simulink model "ADU_Integration_R2014a_simulation"  (R2014a)
settings: Solver=FixedStepDiscrete  StartTime=285  StopTime=300  FixedStep=0.01  RelTol=1e-3
PostLoadFcn:
  | , if any(exist('dsrtsu_mdlpostloadfcn', 'file') == [2, 3, 6]), try dsrtsu_mdlpostloadfcn('Execute', bdroot); catch fprintf('Error in PostLoadFcn (dsrtsu_mdlpostloadfcn) for model "%s":\n %s\n', bdroot, lasterr); end, end,
InitFcn:
  | load 'data/chi2_dat';
  | load 'data/Line_struct';
  | load 'data/innerLNM_1';
  | load 'data/middleLNM_2';
  | load 'data/outerLNM_1';
  | load 'data/landmarks_patac_schimmel_ccw';
  | load 'data/patac_navi_array';
  | load 'data/sensor';
  | load 'data/map_struct';
  | addpath map_src
  | Integration_Parameter;
  | load 'TestData_001';
values from neighbouring files (symbols this model uses):
  TestData_001 =     [TestData_001.mat]
undefined symbols (not defined in the file or in its folder): chi2_dat, innerLNM_1, landmarks_patac_schimmel_ccw, middleLNM_2, outerLNM_1, patac_navi_array
libraries: simulink x36, rtican x1
(part 3 of 22)

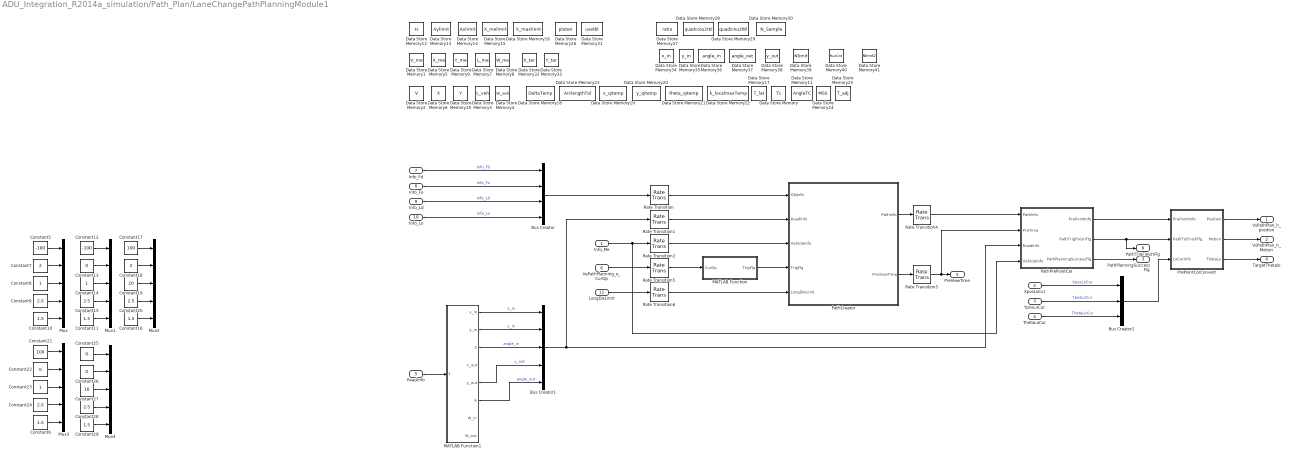
== system ADU_Integration_R2014a_simulation/Path_Plan/LaneChangePathPlanningModule1 ==
  Info_Me : Inport
  XposLoCur : Inport  Port=2
  YposLoCur : Inport  Port=3
  ThetaLoCur : Inport  Port=4
  RoadInfo : Inport  Port=5
  VePathPlanning_e_CurOp : Inport  Port=6
  Info_Fd : Inport  Port=7
  Info_Fo : Inport  Port=8
  Info_Ld : Inport  Port=9
  Info_Lo : Inport  Port=10
  LongDisLimit : Inport  Port=11
  Bus Creator : BusCreator  Inputs=4
  Bus Creator1 : BusCreator  Inputs=5
  Bus Creator2 : BusCreator  Inputs=3
  Constant{6,10..11,16,29} (5 alike) : Constant  Value=1.5
  Constant12 : Constant  Value=-100
  Constant{13,22,25..26} (4 alike) : Constant  Value=0
  Constant14 : Constant
  Constant{9,15,20,24,28} (5 alike) : Constant  Value=2.5
  Constant17 : Constant  Value=100
  Constant18 : Constant  Value=2
  Constant19 : Constant  Value=20
  Constant21 : Constant  Value=100
  Constant23 : Constant
  Constant27 : Constant  Value=10
  Constant5 : Constant  Value=-100
  Constant7 : Constant  Value=2
  Constant8 : Constant
  Data Store Memory : DataStoreMemory  DataStoreName=Tc  ReadBeforeWriteMsg=warning  WriteAfterWriteMsg=warning  WriteAfterReadMsg=warning  InitialValue=[0 0 0 0]  ShowAdditionalParam=off  OutDataTypeStr=double
  Data Store Memory1 : DataStoreMemory  DataStoreName=V_me  ReadBeforeWriteMsg=warning  WriteAfterWriteMsg=warning  WriteAfterReadMsg=warning  ShowAdditionalParam=off  OutDataTypeStr=double
  Data Store Memory10 : DataStoreMemory  DataStoreName=Y  ReadBeforeWriteMsg=warning  WriteAfterWriteMsg=warning  WriteAfterReadMsg=warning  InitialValue=[0 0 0 0]  ShowAdditionalParam=off  OutDataTypeStr=double
  Data Store Memory11 : DataStoreMemory  DataStoreName=AngleTC  ReadBeforeWriteMsg=warning  WriteAfterWriteMsg=warning  WriteAfterReadMsg=warning  InitialValue=[0 0 0 0]  ShowAdditionalParam=off  OutDataTypeStr=double
  Data Store Memory12 : DataStoreMemory  DataStoreName=H  ReadBeforeWriteMsg=warning  WriteAfterWriteMsg=warning  WriteAfterReadMsg=warning  ShowAdditionalParam=off  OutDataTypeStr=double
  Data Store Memory13 : DataStoreMemory  DataStoreName=Aylimit  ReadBeforeWriteMsg=warning  WriteAfterWriteMsg=warning  WriteAfterReadMsg=warning  ShowAdditionalParam=off  OutDataTypeStr=double
  Data Store Memory14 : DataStoreMemory  DataStoreName=Axlimit  ReadBeforeWriteMsg=warning  WriteAfterWriteMsg=warning  WriteAfterReadMsg=warning  ShowAdditionalParam=off  OutDataTypeStr=double
  Data Store Memory15 : DataStoreMemory  DataStoreName=X_melimit  ReadBeforeWriteMsg=warning  WriteAfterWriteMsg=warning  WriteAfterReadMsg=warning  ShowAdditionalParam=off  OutDataTypeStr=double
  Data Store Memory16 : DataStoreMemory  DataStoreName=k_maxlimit  ReadBeforeWriteMsg=warning  WriteAfterWriteMsg=warning  WriteAfterReadMsg=warning  ShowAdditionalParam=off  OutDataTypeStr=double
  Data Store Memory17 : DataStoreMemory  DataStoreName=T_lat  ReadBeforeWriteMsg=warning  WriteAfterWriteMsg=warning  WriteAfterReadMsg=warning  ShowAdditionalParam=off  OutDataTypeStr=double
  Data Store Memory18 : DataStoreMemory  DataStoreName=DeltaTemp  ReadBeforeWriteMsg=warning  WriteAfterWriteMsg=warning  WriteAfterReadMsg=warning  InitialValue=[0 0]  ShowAdditionalParam=off  OutDataTypeStr=double
  Data Store Memory19 : DataStoreMemory  DataStoreName=x_qitemp  ReadBeforeWriteMsg=warning  WriteAfterWriteMsg=warning  WriteAfterReadMsg=warning  ShowAdditionalParam=off  OutDataTypeStr=double
  Data Store Memory2 : DataStoreMemory  DataStoreName=V  ReadBeforeWriteMsg=warning  WriteAfterWriteMsg=warning  WriteAfterReadMsg=warning  InitialValue=[0 0 0 0]  ShowAdditionalParam=off  OutDataTypeStr=double
  Data Store Memory20 : DataStoreMemory  DataStoreName=y_qitemp  ReadBeforeWriteMsg=warning  WriteAfterWriteMsg=warning  WriteAfterReadMsg=warning  ShowAdditionalParam=off  OutDataTypeStr=double
  Data Store Memory21 : DataStoreMemory  DataStoreName=theta_qitemp  ReadBeforeWriteMsg=warning  WriteAfterWriteMsg=warning  WriteAfterReadMsg=warning  ShowAdditionalParam=off  OutDataTypeStr=double
  Data Store Memory22 : DataStoreMemory  DataStoreName=k_localmaxTemp  ReadBeforeWriteMsg=warning  WriteAfterWriteMsg=warning  WriteAfterReadMsg=warning  InitialValue=[0 0]  ShowAdditionalParam=off  OutDataTypeStr=double
  Data Store Memory23 : DataStoreMemory  DataStoreName=ArclengthTol  ReadBeforeWriteMsg=warning  WriteAfterWriteMsg=warning  WriteAfterReadMsg=warning  InitialValue=[0 0]  ShowAdditionalParam=off  OutDataTypeStr=double
  Data Store Memory24 : DataStoreMemory  DataStoreName=MSS  ReadBeforeWriteMsg=warning  WriteAfterWriteMsg=warning  WriteAfterReadMsg=warning  InitialValue=[0 0 0 0]  ShowAdditionalParam=off  OutDataTypeStr=double
  Data Store Memory25 : DataStoreMemory  DataStoreName=T_adj  ReadBeforeWriteMsg=warning  WriteAfterWriteMsg=warning  WriteAfterReadMsg=warning  ShowAdditionalParam=off  OutDataTypeStr=double
  Data Store Memory26 : DataStoreMemory  DataStoreName=ploten  ReadBeforeWriteMsg=warning  WriteAfterWriteMsg=warning  WriteAfterReadMsg=warning  ShowAdditionalParam=off  OutDataTypeStr=double
  Data Store Memory27 : DataStoreMemory  DataStoreName=ratio  ReadBeforeWriteMsg=warning  WriteAfterWriteMsg=warning  WriteAfterReadMsg=warning  ShowAdditionalParam=off  OutDataTypeStr=double
  Data Store Memory28 : DataStoreMemory  DataStoreName=quadcosu2tbl  ReadBeforeWriteMsg=warning  WriteAfterWriteMsg=warning  WriteAfterReadMsg=warning  InitialValue=zeros(1,356)  ShowAdditionalParam=off  OutDataTypeStr=double
  Data Store Memory29 : DataStoreMemory  DataStoreName=quadsinu2tbl  ReadBeforeWriteMsg=warning  WriteAfterWriteMsg=warning  WriteAfterReadMsg=warning  InitialValue=zeros(1,356)  ShowAdditionalParam=off  OutDataTypeStr=double
  Data Store Memory3 : DataStoreMemory  DataStoreName=L_veh  ReadBeforeWriteMsg=warning  WriteAfterWriteMsg=warning  WriteAfterReadMsg=warning  InitialValue=[0 0 0 0]  ShowAdditionalParam=off  OutDataTypeStr=double
  Data Store Memory30 : DataStoreMemory  DataStoreName=N_Sample  ReadBeforeWriteMsg=warning  WriteAfterWriteMsg=warning  WriteAfterReadMsg=warning  ShowAdditionalParam=off  OutDataTypeStr=double
  Data Store Memory31 : DataStoreMemory  DataStoreName=usetbl  ReadBeforeWriteMsg=warning  WriteAfterWriteMsg=warning  WriteAfterReadMsg=warning  ShowAdditionalParam=off  OutDataTypeStr=double
  Data Store Memory32 : DataStoreMemory  DataStoreName=X_tar  ReadBeforeWriteMsg=warning  WriteAfterWriteMsg=warning  WriteAfterReadMsg=warning  ShowAdditionalParam=off  OutDataTypeStr=double
  Data Store Memory33 : DataStoreMemory  DataStoreName=Y_tar  ReadBeforeWriteMsg=warning  WriteAfterWriteMsg=warning  WriteAfterReadMsg=warning  ShowAdditionalParam=off  OutDataTypeStr=double
  Data Store Memory34 : DataStoreMemory  DataStoreName=x_in  ReadBeforeWriteMsg=warning  WriteAfterWriteMsg=warning  WriteAfterReadMsg=warning  ShowAdditionalParam=off  OutDataTypeStr=double
  Data Store Memory35 : DataStoreMemory  DataStoreName=y_in  ReadBeforeWriteMsg=warning  WriteAfterWriteMsg=warning  WriteAfterReadMsg=warning  ShowAdditionalParam=off  OutDataTypeStr=double
  Data Store Memory36 : DataStoreMemory  DataStoreName=angle_in  ReadBeforeWriteMsg=warning  WriteAfterWriteMsg=warning  WriteAfterReadMsg=warning  ShowAdditionalParam=off  OutDataTypeStr=double
  Data Store Memory37 : DataStoreMemory  DataStoreName=angle_out  ReadBeforeWriteMsg=warning  WriteAfterWriteMsg=warning  WriteAfterReadMsg=warning  ShowAdditionalParam=off  OutDataTypeStr=double
  Data Store Memory38 : DataStoreMemory  DataStoreName=y_out  ReadBeforeWriteMsg=warning  WriteAfterWriteMsg=warning  WriteAfterReadMsg=warning  ShowAdditionalParam=off  OutDataTypeStr=double
  Data Store Memory39 : DataStoreMemory  DataStoreName=Nlimit  ReadBeforeWriteMsg=warning  WriteAfterWriteMsg=warning  WriteAfterReadMsg=warning  ShowAdditionalParam=off  OutDataTypeStr=double
  Data Store Memory4 : DataStoreMemory  DataStoreName=W_veh  ReadBeforeWriteMsg=warning  WriteAfterWriteMsg=warning  WriteAfterReadMsg=warning  InitialValue=[0 0 0 0]  ShowAdditionalParam=off  OutDataTypeStr=double
  Data Store Memory40 : DataStoreMemory  DataStoreName=RunCnt  ReadBeforeWriteMsg=warning  WriteAfterWriteMsg=warning  WriteAfterReadMsg=warning  InitialValue=[0 0 0 0]  ShowAdditionalParam=off  OutDataTypeStr=double
  Data Store Memory41 : DataStoreMemory  DataStoreName=Nlimit2  ReadBeforeWriteMsg=warning  WriteAfterWriteMsg=warning  WriteAfterReadMsg=warning  ShowAdditionalParam=off  OutDataTypeStr=double
  Data Store Memory5 : DataStoreMemory  DataStoreName=X_me  ReadBeforeWriteMsg=warning  WriteAfterWriteMsg=warning  WriteAfterReadMsg=warning  ShowAdditionalParam=off  OutDataTypeStr=double
  Data Store Memory6 : DataStoreMemory  DataStoreName=X  ReadBeforeWriteMsg=warning  WriteAfterWriteMsg=warning  WriteAfterReadMsg=warning  InitialValue=[0 0 0 0]  ShowAdditionalParam=off  OutDataTypeStr=double
  Data Store Memory7 : DataStoreMemory  DataStoreName=L_me  ReadBeforeWriteMsg=warning  WriteAfterWriteMsg=warning  WriteAfterReadMsg=warning  ShowAdditionalParam=off  OutDataTypeStr=double
  Data Store Memory8 : DataStoreMemory  DataStoreName=W_me  ReadBeforeWriteMsg=warning  WriteAfterWriteMsg=warning  WriteAfterReadMsg=warning  ShowAdditionalParam=off  OutDataTypeStr=double
  Data Store Memory9 : DataStoreMemory  DataStoreName=Y_me  ReadBeforeWriteMsg=warning  WriteAfterWriteMsg=warning  WriteAfterReadMsg=warning  ShowAdditionalParam=off  OutDataTypeStr=double
  MATLAB Function : MATLAB Function  TreatAsAtomicUnit=on
      settings: PermitHierarchicalResolution=ParametersOnly
  MATLAB Function1 : MATLAB Function  TreatAsAtomicUnit=on
      settings: PermitHierarchicalResolution=ParametersOnly
  Mux{,1..4} (5 alike) : Mux  Inputs=5
  PathCreator : Subsystem  TreatAsAtomicUnit=on  SystemSampleTime=0.02
  PathPrePointCal : Subsystem  TreatAsAtomicUnit=on
  PrePointCorConvert : Subsystem  TreatAsAtomicUnit=on
  Rate Transition{,1..2,5..6} (5 alike) : RateTransition  OutPortSampleTime=0.02
  Rate Transition3 : RateTransition  OutPortSampleTime=0.01
  Rate Transition4 : RateTransition  OutPortSampleTime=0.01
  VsPathPlan_h_position : Outport
  VsPathPlan_h_Motion : Outport  Port=2
  PathPlanningSuccessFlg : Outport  Port=3
  TargetThetalo : Outport  Port=4
  PreViewTime : Outport  Port=5
  PathTrigFinishFlg : Outport  Port=6
  wires:
  MATLAB Function/1(TrigFlg) -> PathCreator/4(TrigFlg)
  Rate Transition5/1 -> MATLAB Function/1(CurOp)
  VePathPlanning_e_CurOp/1 -> Rate Transition5/1
  Rate Transition3/1 -> PreViewTime/1, PathPrePointCal/2(PreTime)
  PathPrePointCal/2(PathTrigFinishFlg) -> PrePointCorConvert/2(PathTrjFinishFlg), PathTrigFinishFlg/1
  PathCreator/2(PreViewTime) -> Rate Transition3/1
  PathPrePointCal/3(PathPlanningSuccessFlg) -> PathPlanningSuccessFlg/1
  Rate Transition4/1 -> PathPrePointCal/1(PathInfo)
  Rate Transition2/1 -> PathCreator/3(VehicleInfo)
  PathCreator/1(PathInfo) -> Rate Transition4/1
  Rate Transition1/1 -> PathCreator/2(RoadInfo)
  Rate Transition/1 -> PathCreator/1(ObjInfo)
  PrePointCorConvert/3(ThetaLo) -> TargetThetalo/1
  PrePointCorConvert/2(Motion) -> VsPathPlan_h_Motion/1
  PrePointCorConvert/1(Position) -> VsPathPlan_h_position/1
  Bus Creator2/1 -> PrePointCorConvert/3(LoCorInfo)
  PathPrePointCal/1(PrePointInfo) -> PrePointCorConvert/1(PrePointInfo)
  ThetaLoCur/1 -> Bus Creator2/3  "ThetaLoCur"
  YposLoCur/1 -> Bus Creator2/2  "YposLoCur"
  XposLoCur/1 -> Bus Creator2/1  "XposLoCur"
  Bus Creator1/1 -> Rate Transition1/1, PathPrePointCal/3(RoadInfo)
  MATLAB Function1/6(angle_out) -> Bus Creator1/5  "angle_out"
  MATLAB Function1/5(y_out) -> Bus Creator1/4  "y_out"
  MATLAB Function1/3(angle_in) -> Bus Creator1/3  "angle_in"
  MATLAB Function1/2(y_in) -> Bus Creator1/2  "y_in"
  MATLAB Function1/1(x_in) -> Bus Creator1/1  "x_in"
  Bus Creator/1 -> Rate Transition/1
  Info_Lo/1 -> Bus Creator/4  "Info_Lo"
  Info_Ld/1 -> Bus Creator/3  "Info_Ld"
  Info_Fo/1 -> Bus Creator/2  "Info_Fo"
  Info_Fd/1 -> Bus Creator/1  "Info_Fd"
  Info_Me/1 -> PathPrePointCal/4(VehicleInfo), Rate Transition2/1
  Constant25/1 -> Mux4/1
  Constant21/1 -> Mux3/1
  Constant27/1 -> Mux4/3
  Constant29/1 -> Mux4/5
  Constant28/1 -> Mux4/4
  Constant26/1 -> Mux4/2
  Constant23/1 -> Mux3/3
  Constant6/1 -> Mux3/5
  Constant24/1 -> Mux3/4
  Constant22/1 -> Mux3/2
  Constant5/1 -> Mux/1
  Constant19/1 -> Mux2/3
  Constant16/1 -> Mux2/5
  Constant20/1 -> Mux2/4
  Constant18/1 -> Mux2/2
  Constant17/1 -> Mux2/1
  Constant14/1 -> Mux1/3
  Constant11/1 -> Mux1/5
  Constant15/1 -> Mux1/4
  Constant13/1 -> Mux1/2
  Constant12/1 -> Mux1/1
  Constant8/1 -> Mux/3
  Constant10/1 -> Mux/5
  Constant9/1 -> Mux/4
  Constant7/1 -> Mux/2
  RoadInfo/1 -> MATLAB Function1/1(RoadInfo)
  LongDisLimit/1 -> Rate Transition6/1
  Rate Transition6/1 -> PathCreator/5(LongDisLimit)

== system ADU_Integration_R2014a_simulation/Path_Plan/PathArbModule ==
  VsPathPlan_h_InterSecposition : Inport
  VsPathPlan_h_InterSecMotion : Inport  Port=2
  VePathPlan_e_InterPPSucFlg : Inport  Port=3
  TargetThetaLoInter : Inport  Port=4
  PreviewTimeInter : Inport  Port=5
  PathTrigFinishFlgInter : Inport  Port=6
  VsPathPlan_h_LCposition : Inport  Port=7
  VsPathPlan_h_LCMotion : Inport  Port=8
  VePathPlan_e_LCPPSucFlg : Inport  Port=9
  TargetThetaLoLC : Inport  Port=10
  PreviewTimeLC : Inport  Port=11
  PathTrigFinishFlgLC : Inport  Port=12
  VePathPlan_e_OutputSelection : Inport  Port=13
  Bus Creator : BusCreator  Inputs=6
  Bus Creator1 : BusCreator  Inputs=6
  Bus Selector : BusSelector  OutputSignals=VsPathPlan_h_position,VsPathPlan_h_Motion,VePathPlan_e_PPSucFlg,TargetThetaLo,PreviewTime,PathTrigFinishFlg
  Switch : Switch  Threshold=0.5
  VsPathPlan_h_position : Outport
  VsPathPlan_h_Motion : Outport  Port=2
  VePathPlan_b_InChargFlg : Outport  Port=3
  TargetThetaLo : Outport  Port=4
  PreviewTime : Outport  Port=5
  PathTrigFinishFlg : Outport  Port=6
  wires:
  Bus Selector/6 -> PathTrigFinishFlg/1  "<PathTrigFinishFlg>"
  PathTrigFinishFlgInter/1 -> Bus Creator1/6  "PathTrigFinishFlg"
  PathTrigFinishFlgLC/1 -> Bus Creator/6  "PathTrigFinishFlg"
  VePathPlan_e_OutputSelection/1 -> Switch/2
  PreviewTimeLC/1 -> Bus Creator/5  "PreviewTime"
  PreviewTimeInter/1 -> Bus Creator1/5  "PreviewTime"
  Bus Selector/1 -> VsPathPlan_h_position/1  "<VsPathPlan_h_position>"
  Bus Selector/2 -> VsPathPlan_h_Motion/1  "<VsPathPlan_h_Motion>"
  Bus Selector/3 -> VePathPlan_b_InChargFlg/1  "<VePathPlan_e_PPSucFlg>"
  Bus Selector/4 -> TargetThetaLo/1  "<TargetThetaLo>"
  Bus Selector/5 -> PreviewTime/1  "<PreviewTime>"
  Switch/1 -> Bus Selector/1
  Bus Creator1/1 -> Switch/3
  VsPathPlan_h_InterSecposition/1 -> Bus Creator1/1  "VsPathPlan_h_position"
  VsPathPlan_h_InterSecMotion/1 -> Bus Creator1/2  "VsPathPlan_h_Motion"
  VePathPlan_e_InterPPSucFlg/1 -> Bus Creator1/3  "VePathPlan_e_PPSucFlg"
  TargetThetaLoInter/1 -> Bus Creator1/4  "TargetThetaLo"
  Bus Creator/1 -> Switch/1
  VsPathPlan_h_LCposition/1 -> Bus Creator/1  "VsPathPlan_h_position"
  VsPathPlan_h_LCMotion/1 -> Bus Creator/2  "VsPathPlan_h_Motion"
  VePathPlan_e_LCPPSucFlg/1 -> Bus Creator/3  "VePathPlan_e_PPSucFlg"
  TargetThetaLoLC/1 -> Bus Creator/4  "TargetThetaLo"

== system ADU_Integration_R2014a_simulation/Path_Plan/SceneSelectionModule ==
  Sur_LandmarkIdList : Inport
  Veh_State : Inport  Port=2
  Object_Info : Inport  Port=3
  Sur_ObjectId_List : Inport  Port=4
  Landmark_Info : Inport  Port=5
  Navi_LandmarkIdList : Inport  Port=6
  EgoLane_Index : Inport  Port=7
  OperationFinishFlg : Inport  Port=8
  ObjSelect : MATLAB Function  TreatAsAtomicUnit=on
      settings: PermitHierarchicalResolution=ParametersOnly
  OpSchedule : MATLAB Function  TreatAsAtomicUnit=on
      settings: PermitHierarchicalResolution=ParametersOnly
  Info_Me : Outport
  Info_Fd : Outport  Port=2
  Info_Fo : Outport  Port=3
  Info_Ld : Outport  Port=4
  Info_Lo : Outport  Port=5
  CurOp : Outport  Port=6
  LongDisLimit : Outport  Port=7
  RoadInfo : Outport  Port=8
  wires:
  OpSchedule/2(OperationLongDislimit) -> LongDisLimit/1
  OperationFinishFlg/1 -> OpSchedule/1(OperationFinishFlg)
  OpSchedule/1(Curoperation) -> CurOp/1
  ObjSelect/1(Info_Fd) -> Info_Fd/1, OpSchedule/6(Info_Fd)
  ObjSelect/2(Info_Fo) -> Info_Fo/1, OpSchedule/7(Info_Fo)
  ObjSelect/4(Info_Lo) -> Info_Lo/1, OpSchedule/9(Info_Lo)
  ObjSelect/3(Info_Ld) -> Info_Ld/1, OpSchedule/8(Info_Ld)
  ObjSelect/5(Info_Me) -> Info_Me/1, OpSchedule/10(Info_Me)
  Object_Info/1 -> ObjSelect/4(Object_Info)
  Veh_State/1 -> ObjSelect/2(Veh_State)
  Sur_ObjectId_List/1 -> ObjSelect/3(Sur_ObjectId_List)
  EgoLane_Index/1 -> OpSchedule/5(EgoLane_Index), ObjSelect/1(EgoLane_Index)
  Landmark_Info/1 -> OpSchedule/2(Landmark_Info)
  Sur_LandmarkIdList/1 -> OpSchedule/3(Sur_LandmarkIdList)
  Navi_LandmarkIdList/1 -> OpSchedule/4(Navi_LandmarkIdList)
  OpSchedule/4(RoadInfo) -> RoadInfo/1

== system ADU_Integration_R2014a_simulation/Fusion_Model/Fusion_Block/Fus_Header_Gen ==
  Target_Num : Inport
  Bus Creator1 : BusCreator  Inputs=7
  CameraValid : Constant
  ESRValid : Constant
  LFSRRValid : Constant
  LRSRRValid1 : Constant
  RFSRRValid1 : Constant
  RRSRRValid2 : Constant
  Fus_Header : Outport
  wires:
  ESRValid/1 -> Bus Creator1/2  "ESRValid"
  LFSRRValid/1 -> Bus Creator1/3  "LFSRRValid"
  CameraValid/1 -> Bus Creator1/1  "CameraValid"
  RFSRRValid1/1 -> Bus Creator1/4  "RFSRRValid"
  RRSRRValid2/1 -> Bus Creator1/6  "RRSRRValid"
  Bus Creator1/1 -> Fus_Header/1
  LRSRRValid1/1 -> Bus Creator1/5  "LRSRRValid"
  Target_Num/1 -> Bus Creator1/7  "Total_Targ_Num"

== system ADU_Integration_R2014a_simulation/Fusion_Model/Fusion_Block/Global_Fusion ==
  From SideFusion : Inport
  From Sensor : Inport  Port=2
  Bus Selector1 : BusSelector  OutputSignals=Vision_Target[25X8]
  Bus Selector2 : BusSelector  OutputSignals=ESR_Data[64X4]
  Curve_Radius[m] : Subsystem
  ESR_TemporalAlig : Stateflow chart  TreatAsAtomicUnit=on
      settings: PermitHierarchicalResolution=ParametersOnly
  Fusion_Center : Stateflow chart  TreatAsAtomicUnit=on
      settings: PermitHierarchicalResolution=ParametersOnly
  Mux : Mux  Inputs=3
  Rate Transition1 : RateTransition  Deterministic=off
  Rate Transition2 : RateTransition  Deterministic=off
  Rate Transition3 : RateTransition  Deterministic=off
  Terminator1 : Terminator
  Terminator3 : Terminator
  GlobalFusOut[127X26] : Outport
  Total_TargetNum : Outport  Port=2
  wires:
  From Sensor/1 -> Bus Selector1/1, Bus Selector2/1
  Bus Selector2/1 -> ESR_TemporalAlig/1(ESR_Input)  "<ESR_Data[64X4]>"
  [ESRcal] -> ESR_TemporalAlig/Trigger
  [CameraCal] -> Mux/1
  [SRRCal] -> Mux/2
  ESR_TemporalAlig/1(ESR_Output) -> Fusion_Center/1(ESRData)
  Fusion_Center/1(FusDataOut) -> GlobalFusOut[127X26]/1
  Fusion_Center/2(Num_Trg) -> Total_TargetNum/1
  Bus Selector1/1 -> Fusion_Center/2(CameraData)  "<Vision_Target[25X8]>"
  From SideFusion/1 -> Fusion_Center/3(SRRData)
  Curve_Radius[m]/1(Curve_Radius[m]) -> Fusion_Center/4(Path_Radius)
  [ESRcal] -> Mux/3
  Mux/1 -> Fusion_Center/Trigger
  Fusion_Center/3(RollCount) -> Terminator3/1
  ESR_TemporalAlig/2(RollCount) -> Terminator1/1
  [CameraTime] -> Rate Transition1/1
  Rate Transition1/1 -> Fusion_Center/7(Camera_RxTime)
  [ESRTime] -> Rate Transition2/1
  Rate Transition2/1 -> Fusion_Center/5(ESR_RxTime)
  [LFSRRTime] -> Rate Transition3/1
  Rate Transition3/1 -> Fusion_Center/6(SRR_RxTime)

== system ADU_Integration_R2014a_simulation/Fusion_Model/Fusion_Block/Side_Fusion ==
  From Sensor : Inport
  Bus Selector2 : BusSelector  OutputSignals=LF_SRR_Data[10X5],RF_SRR_Data[10X5],LR_SRR_Data[10X5],RR_SRR_Data[10X5]
  LF_SRR_CoordinateAlig : Stateflow chart  TreatAsAtomicUnit=on
      settings: PermitHierarchicalResolution=ParametersOnly
  LR_SRR_CoordinateAlig : Stateflow chart  TreatAsAtomicUnit=on
      settings: PermitHierarchicalResolution=ParametersOnly
  Mux : Mux
  RF_SRR_CoordinateAlig : Stateflow chart  TreatAsAtomicUnit=on
      settings: PermitHierarchicalResolution=ParametersOnly
  RR_SRR_CoordinateAlig : Stateflow chart  TreatAsAtomicUnit=on
      settings: PermitHierarchicalResolution=ParametersOnly
  Rate Transition{1..4} (4 alike) : RateTransition  Deterministic=off
  SRR_Data_Out : Stateflow chart  TreatAsAtomicUnit=on
      settings: PermitHierarchicalResolution=ParametersOnly
  Side_Fusion : Stateflow chart  TreatAsAtomicUnit=on
      settings: PermitHierarchicalResolution=ParametersOnly
  SideFus_Output[40X4] : Outport
  SideRadar_RawData[40X4] : Outport  Port=2
  tag scope: SRRCal=global
  wires:
  Bus Selector2/1 -> LF_SRR_CoordinateAlig/1(LFSRR_Input)  "<LF_SRR_Data[10X5]>"
  Bus Selector2/2 -> RF_SRR_CoordinateAlig/1(RFSRR_Input)  "<RF_SRR_Data[10X5]>"
  Bus Selector2/3 -> LR_SRR_CoordinateAlig/1(LRSRR_Input)  "<LR_SRR_Data[10X5]>"
  Bus Selector2/4 -> RR_SRR_CoordinateAlig/1(RRSRR_Input)  "<RR_SRR_Data[10X5]>"
  LF_SRR_CoordinateAlig/1(LFSRR_Output) -> Side_Fusion/1(LFSRR_Input), SRR_Data_Out/1(LFSRR_Input)
  RF_SRR_CoordinateAlig/1(RFSRR_Output) -> Side_Fusion/3(RFSRR_Input), SRR_Data_Out/2(RFSRR_Input)
  LR_SRR_CoordinateAlig/1(LRSRR_Output) -> Side_Fusion/5(LRSRR_Input), SRR_Data_Out/3(LRSRR_Input)
  Side_Fusion/1(SideFusOut) -> SideFus_Output[40X4]/1
  From Sensor/1 -> Bus Selector2/1
  [LFSRRcal] -> LF_SRR_CoordinateAlig/Trigger
  [LRSRRcal] -> LR_SRR_CoordinateAlig/Trigger
  [RRSRRcal] -> RR_SRR_CoordinateAlig/Trigger
  LF_SRR_CoordinateAlig/2(SideFusion()) -> [LFSRRUpdate]
  RF_SRR_CoordinateAlig/2(SideFusion()) -> [RFSRRUpdate]
  LR_SRR_CoordinateAlig/2(SideFusion()) -> [LRSRRUpdate]
  RR_SRR_CoordinateAlig/2(SideFusion()) -> [RRSRRUpdate]
  [LFSRRUpdate] -> Mux/1
  [RFSRRUpdate] -> Mux/2
  [LRSRRUpdate] -> Mux/3
  [RRSRRUpdate] -> Mux/4
  [RFSRRcal] -> RF_SRR_CoordinateAlig/Trigger
  SRR_Data_Out/1(SRR_Data) -> SideRadar_RawData[40X4]/1
  Side_Fusion/2(Global_Fus_Event) -> [SRRCal]
  Mux/1 -> Side_Fusion/Trigger
  Rate Transition2/1 -> Side_Fusion/2(LFSRR_RxTm)
  [LFSRRTime] -> Rate Transition2/1
  Rate Transition1/1 -> Side_Fusion/4(RFSRR_RxTm)
  [RFSRRTime] -> Rate Transition1/1
  Rate Transition3/1 -> Side_Fusion/6(LRSRR_RxTm)
  [LRSRRTime] -> Rate Transition3/1
  Rate Transition4/1 -> Side_Fusion/8(RRSRR_RxTm)
  [RRSRRTime] -> Rate Transition4/1
  RR_SRR_CoordinateAlig/1(RRSRR_Output) -> Side_Fusion/7(RRSRR_Input), SRR_Data_Out/4(RRSRR_Input)

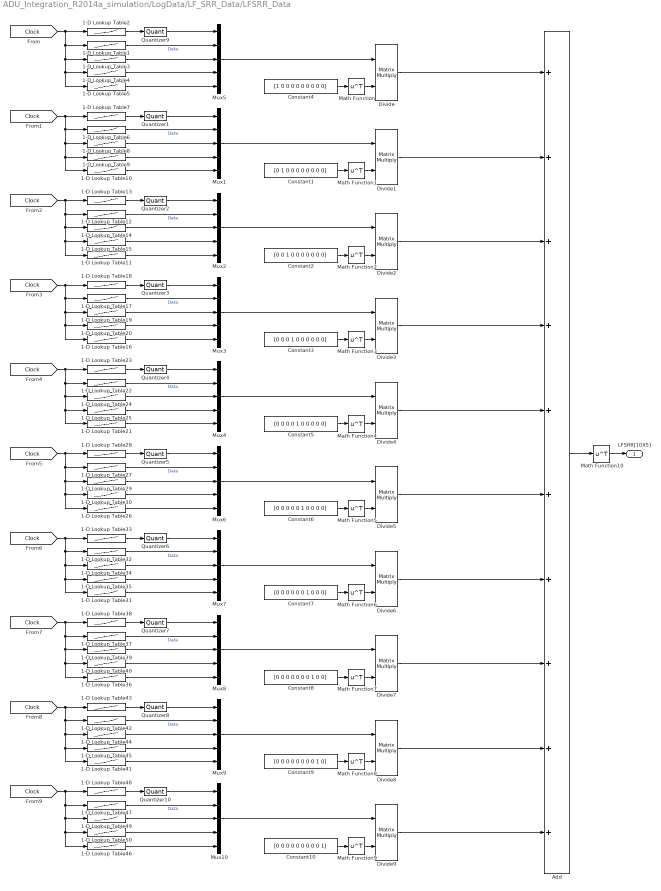
== system ADU_Integration_R2014a_simulation/LogData/LF_SRR_Data/LFSRR_Data ==
  1-D Lookup Table1 : Lookup_n-D  NumberOfTableDimensions=1  BreakpointsForDimension1=TestData_001.X.Data  Table=TestData_001.Y(2+5*0).Data  RndMeth=Simplest  InputSameDT=on
  1-D Lookup Table10 : Lookup_n-D  NumberOfTableDimensions=1  BreakpointsForDimension1=TestData_001.X.Data  Table=TestData_001.Y(5+5*1).Data  RndMeth=Simplest  InputSameDT=on
  1-D Lookup Table11 : Lookup_n-D  NumberOfTableDimensions=1  BreakpointsForDimension1=TestData_001.X.Data  Table=TestData_001.Y(5+5*2).Data  RndMeth=Simplest  InputSameDT=on
  1-D Lookup Table12 : Lookup_n-D  NumberOfTableDimensions=1  BreakpointsForDimension1=TestData_001.X.Data  Table=TestData_001.Y(2+5*2).Data  RndMeth=Simplest  InputSameDT=on
  1-D Lookup Table13 : Lookup_n-D  NumberOfTableDimensions=1  BreakpointsForDimension1=TestData_001.X.Data  Table=TestData_001.Y(1+5*2).Data  RndMeth=Simplest  InputSameDT=on
  1-D Lookup Table14 : Lookup_n-D  NumberOfTableDimensions=1  BreakpointsForDimension1=TestData_001.X.Data  Table=TestData_001.Y(3+5*2).Data  RndMeth=Simplest  InputSameDT=on
  1-D Lookup Table15 : Lookup_n-D  NumberOfTableDimensions=1  BreakpointsForDimension1=TestData_001.X.Data  Table=TestData_001.Y(4+5*2).Data  RndMeth=Simplest  InputSameDT=on
  1-D Lookup Table16 : Lookup_n-D  NumberOfTableDimensions=1  BreakpointsForDimension1=TestData_001.X.Data  Table=TestData_001.Y(5+5*3).Data  RndMeth=Simplest  InputSameDT=on
  1-D Lookup Table17 : Lookup_n-D  NumberOfTableDimensions=1  BreakpointsForDimension1=TestData_001.X.Data  Table=TestData_001.Y(2+5*3).Data  RndMeth=Simplest  InputSameDT=on
  1-D Lookup Table18 : Lookup_n-D  NumberOfTableDimensions=1  BreakpointsForDimension1=TestData_001.X.Data  Table=TestData_001.Y(1+5*3).Data  RndMeth=Simplest  InputSameDT=on
  1-D Lookup Table19 : Lookup_n-D  NumberOfTableDimensions=1  BreakpointsForDimension1=TestData_001.X.Data  Table=TestData_001.Y(3+5*3).Data  RndMeth=Simplest  InputSameDT=on
  1-D Lookup Table2 : Lookup_n-D  NumberOfTableDimensions=1  BreakpointsForDimension1=TestData_001.X.Data  Table=TestData_001.Y(1+5*0).Data  RndMeth=Simplest  InputSameDT=on
  1-D Lookup Table20 : Lookup_n-D  NumberOfTableDimensions=1  BreakpointsForDimension1=TestData_001.X.Data  Table=TestData_001.Y(4+5*3).Data  RndMeth=Simplest  InputSameDT=on
  1-D Lookup Table21 : Lookup_n-D  NumberOfTableDimensions=1  BreakpointsForDimension1=TestData_001.X.Data  Table=TestData_001.Y(5+5*4).Data  RndMeth=Simplest  InputSameDT=on
  1-D Lookup Table22 : Lookup_n-D  NumberOfTableDimensions=1  BreakpointsForDimension1=TestData_001.X.Data  Table=TestData_001.Y(2+5*4).Data  RndMeth=Simplest  InputSameDT=on
  1-D Lookup Table23 : Lookup_n-D  NumberOfTableDimensions=1  BreakpointsForDimension1=TestData_001.X.Data  Table=TestData_001.Y(1+5*4).Data  RndMeth=Simplest  InputSameDT=on
  1-D Lookup Table24 : Lookup_n-D  NumberOfTableDimensions=1  BreakpointsForDimension1=TestData_001.X.Data  Table=TestData_001.Y(3+5*4).Data  RndMeth=Simplest  InputSameDT=on
  1-D Lookup Table25 : Lookup_n-D  NumberOfTableDimensions=1  BreakpointsForDimension1=TestData_001.X.Data  Table=TestData_001.Y(4+5*4).Data  RndMeth=Simplest  InputSameDT=on
  1-D Lookup Table26 : Lookup_n-D  NumberOfTableDimensions=1  BreakpointsForDimension1=TestData_001.X.Data  Table=TestData_001.Y(5+5*5).Data  RndMeth=Simplest  InputSameDT=on
  1-D Lookup Table27 : Lookup_n-D  NumberOfTableDimensions=1  BreakpointsForDimension1=TestData_001.X.Data  Table=TestData_001.Y(2+5*5).Data  RndMeth=Simplest  InputSameDT=on
  1-D Lookup Table28 : Lookup_n-D  NumberOfTableDimensions=1  BreakpointsForDimension1=TestData_001.X.Data  Table=TestData_001.Y(1+5*5).Data  RndMeth=Simplest  InputSameDT=on
  1-D Lookup Table29 : Lookup_n-D  NumberOfTableDimensions=1  BreakpointsForDimension1=TestData_001.X.Data  Table=TestData_001.Y(3+5*5).Data  RndMeth=Simplest  InputSameDT=on
  1-D Lookup Table3 : Lookup_n-D  NumberOfTableDimensions=1  BreakpointsForDimension1=TestData_001.X.Data  Table=TestData_001.Y(3+5*0).Data  RndMeth=Simplest  InputSameDT=on
  1-D Lookup Table30 : Lookup_n-D  NumberOfTableDimensions=1  BreakpointsForDimension1=TestData_001.X.Data  Table=TestData_001.Y(4+5*5).Data  RndMeth=Simplest  InputSameDT=on
  1-D Lookup Table31 : Lookup_n-D  NumberOfTableDimensions=1  BreakpointsForDimension1=TestData_001.X.Data  Table=TestData_001.Y(5+5*6).Data  RndMeth=Simplest  InputSameDT=on
  1-D Lookup Table32 : Lookup_n-D  NumberOfTableDimensions=1  BreakpointsForDimension1=TestData_001.X.Data  Table=TestData_001.Y(2+5*6).Data  RndMeth=Simplest  InputSameDT=on
  1-D Lookup Table33 : Lookup_n-D  NumberOfTableDimensions=1  BreakpointsForDimension1=TestData_001.X.Data  Table=TestData_001.Y(1+5*6).Data  RndMeth=Simplest  InputSameDT=on
  1-D Lookup Table34 : Lookup_n-D  NumberOfTableDimensions=1  BreakpointsForDimension1=TestData_001.X.Data  Table=TestData_001.Y(3+5*6).Data  RndMeth=Simplest  InputSameDT=on
  1-D Lookup Table35 : Lookup_n-D  NumberOfTableDimensions=1  BreakpointsForDimension1=TestData_001.X.Data  Table=TestData_001.Y(4+5*6).Data  RndMeth=Simplest  InputSameDT=on
  1-D Lookup Table36 : Lookup_n-D  NumberOfTableDimensions=1  BreakpointsForDimension1=TestData_001.X.Data  Table=TestData_001.Y(5+5*7).Data  RndMeth=Simplest  InputSameDT=on
  1-D Lookup Table37 : Lookup_n-D  NumberOfTableDimensions=1  BreakpointsForDimension1=TestData_001.X.Data  Table=TestData_001.Y(2+5*7).Data  RndMeth=Simplest  InputSameDT=on
  1-D Lookup Table38 : Lookup_n-D  NumberOfTableDimensions=1  BreakpointsForDimension1=TestData_001.X.Data  Table=TestData_001.Y(1+5*7).Data  RndMeth=Simplest  InputSameDT=on
  1-D Lookup Table39 : Lookup_n-D  NumberOfTableDimensions=1  BreakpointsForDimension1=TestData_001.X.Data  Table=TestData_001.Y(3+5*7).Data  RndMeth=Simplest  InputSameDT=on
  1-D Lookup Table4 : Lookup_n-D  NumberOfTableDimensions=1  BreakpointsForDimension1=TestData_001.X.Data  Table=TestData_001.Y(4+5*0).Data  RndMeth=Simplest  InputSameDT=on
  1-D Lookup Table40 : Lookup_n-D  NumberOfTableDimensions=1  BreakpointsForDimension1=TestData_001.X.Data  Table=TestData_001.Y(4+5*7).Data  RndMeth=Simplest  InputSameDT=on
  1-D Lookup Table41 : Lookup_n-D  NumberOfTableDimensions=1  BreakpointsForDimension1=TestData_001.X.Data  Table=TestData_001.Y(5+5*8).Data  RndMeth=Simplest  InputSameDT=on
  1-D Lookup Table42 : Lookup_n-D  NumberOfTableDimensions=1  BreakpointsForDimension1=TestData_001.X.Data  Table=TestData_001.Y(2+5*8).Data  RndMeth=Simplest  InputSameDT=on
  1-D Lookup Table43 : Lookup_n-D  NumberOfTableDimensions=1  BreakpointsForDimension1=TestData_001.X.Data  Table=TestData_001.Y(1+5*8).Data  RndMeth=Simplest  InputSameDT=on
  1-D Lookup Table44 : Lookup_n-D  NumberOfTableDimensions=1  BreakpointsForDimension1=TestData_001.X.Data  Table=TestData_001.Y(3+5*8).Data  RndMeth=Simplest  InputSameDT=on
  1-D Lookup Table45 : Lookup_n-D  NumberOfTableDimensions=1  BreakpointsForDimension1=TestData_001.X.Data  Table=TestData_001.Y(4+5*8).Data  RndMeth=Simplest  InputSameDT=on
  1-D Lookup Table46 : Lookup_n-D  NumberOfTableDimensions=1  BreakpointsForDimension1=TestData_001.X.Data  Table=TestData_001.Y(5+5*9).Data  RndMeth=Simplest  InputSameDT=on
  1-D Lookup Table47 : Lookup_n-D  NumberOfTableDimensions=1  BreakpointsForDimension1=TestData_001.X.Data  Table=TestData_001.Y(2+5*9).Data  RndMeth=Simplest  InputSameDT=on
  1-D Lookup Table48 : Lookup_n-D  NumberOfTableDimensions=1  BreakpointsForDimension1=TestData_001.X.Data  Table=TestData_001.Y(1+5*9).Data  RndMeth=Simplest  InputSameDT=on
  1-D Lookup Table49 : Lookup_n-D  NumberOfTableDimensions=1  BreakpointsForDimension1=TestData_001.X.Data  Table=TestData_001.Y(3+5*9).Data  RndMeth=Simplest  InputSameDT=on
  1-D Lookup Table5 : Lookup_n-D  NumberOfTableDimensions=1  BreakpointsForDimension1=TestData_001.X.Data  Table=TestData_001.Y(5+5*0).Data  RndMeth=Simplest  InputSameDT=on
  1-D Lookup Table50 : Lookup_n-D  NumberOfTableDimensions=1  BreakpointsForDimension1=TestData_001.X.Data  Table=TestData_001.Y(4+5*9).Data  RndMeth=Simplest  InputSameDT=on
  1-D Lookup Table6 : Lookup_n-D  NumberOfTableDimensions=1  BreakpointsForDimension1=TestData_001.X.Data  Table=TestData_001.Y(2+5*1).Data  RndMeth=Simplest  InputSameDT=on
  1-D Lookup Table7 : Lookup_n-D  NumberOfTableDimensions=1  BreakpointsForDimension1=TestData_001.X.Data  Table=TestData_001.Y(1+5*1).Data  RndMeth=Simplest  InputSameDT=on
  1-D Lookup Table8 : Lookup_n-D  NumberOfTableDimensions=1  BreakpointsForDimension1=TestData_001.X.Data  Table=TestData_001.Y(3+5*1).Data  RndMeth=Simplest  InputSameDT=on
  1-D Lookup Table9 : Lookup_n-D  NumberOfTableDimensions=1  BreakpointsForDimension1=TestData_001.X.Data  Table=TestData_001.Y(4+5*1).Data  RndMeth=Simplest  InputSameDT=on
  Add : Sum  Inputs=++++++++++
  Constant1 : Constant  Value=[0 1 0 0 0 0 0 0 0 0]
  Constant10 : Constant  Value=[0 0 0 0 0 0 0 0 0 1]
  Constant2 : Constant  Value=[0 0 1 0 0 0 0 0 0 0]
  Constant3 : Constant  Value=[0 0 0 1 0 0 0 0 0 0]
  Constant4 : Constant  Value=[1 0 0 0 0 0 0 0 0 0]
  Constant5 : Constant  Value=[0 0 0 0 1 0 0 0 0 0]
  Constant6 : Constant  Value=[0 0 0 0 0 1 0 0 0 0]
  Constant7 : Constant  Value=[0 0 0 0 0 0 1 0 0 0]
  Constant8 : Constant  Value=[0 0 0 0 0 0 0 1 0 0]
  Constant9 : Constant  Value=[0 0 0 0 0 0 0 0 1 0]
  Divide{,1..9} (10 alike) : Product  Inputs=**  Multiplication=Matrix(*)
  Math Function{,1..10} (11 alike) : Math  Operator=transpose  SaturateOnIntegerOverflow=on
  Mux{1..10} (10 alike) : Mux  Inputs=5
  Quantizer{1..10} (10 alike) : Quantizer  QuantizationInterval=1
  LFSRR[10X5] : Outport
  wires:
  Mux5/1 -> Divide/1
  Constant4/1 -> Math Function/1
  Math Function/1 -> Divide/2
  Divide/1 -> Add/1
  Math Function4/1 -> Divide4/2
  Math Function3/1 -> Divide3/2
  Divide3/1 -> Add/4
  Constant9/1 -> Math Function8/1
  Math Function6/1 -> Divide6/2
  Divide1/1 -> Add/2
  Divide4/1 -> Add/5
  Quantizer9/1 -> Mux5/1
  Constant7/1 -> Math Function6/1
  Divide2/1 -> Add/3
  Divide9/1 -> Add/10
  Constant3/1 -> Math Function3/1
  Divide5/1 -> Add/6
  Math Function5/1 -> Divide5/2
  1-D Lookup Table4/1 -> Mux5/4
  1-D Lookup Table3/1 -> Mux5/3
  Constant8/1 -> Math Function7/1
  Divide6/1 -> Add/7
  Math Function8/1 -> Divide8/2
  Constant5/1 -> Math Function4/1
  Math Function9/1 -> Divide9/2
  Math Function7/1 -> Divide7/2
  Constant10/1 -> Math Function9/1
  Math Function2/1 -> Divide2/2
  Constant1/1 -> Math Function1/1
  Divide7/1 -> Add/8
  Divide8/1 -> Add/9
  Constant2/1 -> Math Function2/1
  Math Function1/1 -> Divide1/2
  Constant6/1 -> Math Function5/1
  Add/1 -> Math Function10/1
  Math Function10/1 -> LFSRR[10X5]/1
  1-D Lookup Table2/1 -> Quantizer9/1
  [Clock] -> 1-D Lookup Table2/1, 1-D Lookup Table1/1, 1-D Lookup Table4/1, 1-D Lookup Table5/1, 1-D Lookup Table3/1
  1-D Lookup Table1/1 -> Mux5/2  "Data"
  1-D Lookup Table5/1 -> Mux5/5
  Mux1/1 -> Divide1/1
  Quantizer1/1 -> Mux1/1
  1-D Lookup Table9/1 -> Mux1/4
  1-D Lookup Table8/1 -> Mux1/3
  1-D Lookup Table7/1 -> Quantizer1/1
  [Clock] -> 1-D Lookup Table8/1, 1-D Lookup Table9/1, 1-D Lookup Table10/1, 1-D Lookup Table6/1, 1-D Lookup Table7/1
  1-D Lookup Table6/1 -> Mux1/2  "Data"
  1-D Lookup Table10/1 -> Mux1/5
  Mux2/1 -> Divide2/1
  Quantizer2/1 -> Mux2/1
  1-D Lookup Table15/1 -> Mux2/4
  1-D Lookup Table14/1 -> Mux2/3
  1-D Lookup Table13/1 -> Quantizer2/1
  [Clock] -> 1-D Lookup Table13/1, 1-D Lookup Table12/1, 1-D Lookup Table11/1, 1-D Lookup Table15/1, 1-D Lookup Table14/1
  1-D Lookup Table12/1 -> Mux2/2  "Data"
  1-D Lookup Table11/1 -> Mux2/5
  Mux3/1 -> Divide3/1
  Quantizer3/1 -> Mux3/1
  1-D Lookup Table20/1 -> Mux3/4
  1-D Lookup Table19/1 -> Mux3/3
  1-D Lookup Table18/1 -> Quantizer3/1
  [Clock] -> 1-D Lookup Table19/1, 1-D Lookup Table20/1, 1-D Lookup Table16/1, 1-D Lookup Table17/1, 1-D Lookup Table18/1
  1-D Lookup Table17/1 -> Mux3/2  "Data"
  1-D Lookup Table16/1 -> Mux3/5
  Mux4/1 -> Divide4/1
  Quantizer4/1 -> Mux4/1
  1-D Lookup Table25/1 -> Mux4/4
  1-D Lookup Table24/1 -> Mux4/3
  1-D Lookup Table23/1 -> Quantizer4/1
  [Clock] -> 1-D Lookup Table23/1, 1-D Lookup Table22/1, 1-D Lookup Table21/1, 1-D Lookup Table25/1, 1-D Lookup Table24/1
  1-D Lookup Table22/1 -> Mux4/2  "Data"
  1-D Lookup Table21/1 -> Mux4/5
  Mux6/1 -> Divide5/1
  Quantizer5/1 -> Mux6/1
  1-D Lookup Table30/1 -> Mux6/4
  1-D Lookup Table29/1 -> Mux6/3
  1-D Lookup Table28/1 -> Quantizer5/1
  [Clock] -> 1-D Lookup Table29/1, 1-D Lookup Table30/1, 1-D Lookup Table26/1, 1-D Lookup Table27/1, 1-D Lookup Table28/1
  1-D Lookup Table27/1 -> Mux6/2  "Data"
  1-D Lookup Table26/1 -> Mux6/5
  Mux7/1 -> Divide6/1
  Quantizer6/1 -> Mux7/1
  1-D Lookup Table35/1 -> Mux7/4
  1-D Lookup Table34/1 -> Mux7/3
  1-D Lookup Table33/1 -> Quantizer6/1
  [Clock] -> 1-D Lookup Table33/1, 1-D Lookup Table32/1, 1-D Lookup Table35/1, 1-D Lookup Table31/1, 1-D Lookup Table34/1
  1-D Lookup Table32/1 -> Mux7/2  "Data"
  1-D Lookup Table31/1 -> Mux7/5
  Mux8/1 -> Divide7/1
  Quantizer7/1 -> Mux8/1
  1-D Lookup Table40/1 -> Mux8/4
  1-D Lookup Table39/1 -> Mux8/3
  1-D Lookup Table38/1 -> Quantizer7/1
  [Clock] -> 1-D Lookup Table39/1, 1-D Lookup Table36/1, 1-D Lookup Table40/1, 1-D Lookup Table37/1, 1-D Lookup Table38/1
  1-D Lookup Table37/1 -> Mux8/2  "Data"
  1-D Lookup Table36/1 -> Mux8/5
  Mux9/1 -> Divide8/1
  Quantizer8/1 -> Mux9/1
  1-D Lookup Table45/1 -> Mux9/4
  1-D Lookup Table44/1 -> Mux9/3
  1-D Lookup Table43/1 -> Quantizer8/1
  [Clock] -> 1-D Lookup Table43/1, 1-D Lookup Table42/1, 1-D Lookup Table45/1, 1-D Lookup Table41/1, 1-D Lookup Table44/1
  1-D Lookup Table42/1 -> Mux9/2  "Data"
  1-D Lookup Table41/1 -> Mux9/5
  Mux10/1 -> Divide9/1
  Quantizer10/1 -> Mux10/1
  1-D Lookup Table50/1 -> Mux10/4
  1-D Lookup Table49/1 -> Mux10/3
  1-D Lookup Table48/1 -> Quantizer10/1
  [Clock] -> 1-D Lookup Table49/1, 1-D Lookup Table46/1, 1-D Lookup Table50/1, 1-D Lookup Table47/1, 1-D Lookup Table48/1
  1-D Lookup Table47/1 -> Mux10/2  "Data"
  1-D Lookup Table46/1 -> Mux10/5
